simulink model "woutModel"  (R2019b)
settings: Solver=VariableStepAuto  StartTime=0.0  StopTime=10.0  RelTol=1e-3
model workspace (MAT data in the model file):
  I1 = 0.074
  I2 = 0.00012
  L = 0.6
  P1 = 0.4356
  P2 = 0.00372
  P3 = 0.036
  Sig = Simulink.Signal
  Sig.DataType = 'auto'
  Sig.Dimensions = -1
  Sig.DimensionsMode = 'auto'
  Sig.Complexity = 'auto'
  Sig.SampleTime = -1
  Sig.SamplingMode = 'auto'
  b1 = 4.8
  b2 = 0.0002
  c1 = 0.04
  c2 = 0.06
  ddtheta = sym
  ddtheta.s = 'symobj::fromString("eJzNVktv1DAQdjYppRTKHkDlUUSg3HqBHouQUm2ptIeKAxdukZc4W6PESeMsND31yC/gP8FvQlpsJ0u8tuPsIg6NNIpnMpnHN4/EBQAMALj+we6e62ywW/AE1JfLzg+aM9MBW5xoRSGleEqEeOn5IadvCBeR/xUWGE4S5BOYIurPKIp8THxapdnky8ksTatxhEiJY4wKIPscKDY9TudZEik6XTEKfZpkpSK/xYmWUYInwt8d0F73OFFUfqzS4wRDimid22PJxy9J/78B9pBTJyargfKqkTNZsN+cHQWkfwHM5XSSpSpYAsgzWBb4UsTY5dNVzj8lG57Cbyg+7nN6f5kXiAGXkVOMeKogeNraE76ft/a4f489D3ZaM0s2eU4DHAm57HvbYOeMyVygXdp7Mn/X0jCuEssmp1FGSlZubvdFIx8y+l7HACJLzW5zChEDiKILU90+zIRdrc4RLKEhj4Ufz2QrxDGw6NSxJPCqCrPCErPomxBdzGAisJTxdZzmbpLP2WXppd2+OSFZzuY52FvY7LDzqG+O6xwhES3UV5sENZlqPmT+mSUv36C7mPWBYe7k/uJ9NKyX3dHRmMSY4LLqmcdVl6XIT7Jpw9DmT62HmoOIYQTzPKlEDKvukgOjHRzVo9bdK4KyXPOlzUMKuVKw28a/ZFOO5bXC7xli7drR6+Qo9gmr1+mMfAY9Prd7/GiYGHbmsGcX3gRexqfefTiO5V07n1/Lu1bOm8ucGGh5q9jp+7X20YWv2g8Hlvkx7jJYTGnvji0gmSIR+9IuHTR3S78eK/zOmr0j828V/t0N6Im1e6ascqTo8e98z3+I87vHtqgTpleoyMT7q/yP9NVF5rl+17+Io+iODe921XjLUGOt/6S8uvpsU3qmxqP6GBlmRN69L9tY/87uou8bXv8+R1F5jkp4aHn2xjR/++Gn8A82IAgb", 2)'
  ddtheta.digits = 32
  ddtheta1 = sym
  ddtheta1.s = 'symobj::fromString("eJytkEEKwjAQRce2igrudKGrXEFPoODGtSdIyWgjSQqdVMnOU3goT2XSCsZCwYUDjxkmn/zkpwCQANwfvmfpYOjbdgVtpX6ev2evgUmAHHEieTbN+ut8E7ihrAS78kryXCEzXCOxmlAwaRg5XeaXfa21Owg0Vp4kVhB7Jp07s0BRKtHR9L2x0ZMqbWc/CpAVSuaN3xQ+NQsQ2qPTOyU5IbV/W0Yez0j/t8AWgd5Mfgsl3o8DQtgCLV+/AARuPcI=", 2)'
  ddtheta1.digits = 32
  ddtheta2 = sym
  ddtheta2.s = 'symobj::fromString("eJytkEEKwjAQRce2igrudKGrnKEnUHDj2hOkZLSRJIVOqmTnKTyUpzJpBWOh4MKBxwyTT37yUwBIAO4P37N0NPZtu4GuUj8v37PXwCxAjjiRPJt2/XWeB24oa8GuvJa8UMgM10isIRRMGkZOV8Vl32jtDgKNlSeJNcSeSe/OLFBWSvQ0Q29s9aQq29tPAmSFkkXrN4dPLQKE9uj0TklOSN3f1pHHM9L/LbBVYDCT30KJ99OAELZEy/MXBG89w3==", 2)'
  ddtheta2.digits = 32
  dtheta = sym
  dtheta.s = 'symobj::fromString("eJzNV09v0zAUd5qOMQajB9D4M0Rgu+0CHIeQMnVM6mHiwIVb5BKnM0qcLHZh2WlHPgHfCT4TUrGdlDiOnbSIwyI9Je/55ff+v6YuAGAAwPUPfh+6zga/+U9Aebn8+UH1zHXAliBaUEgpnhEpbpy/EfQN4Tz0vsIcw2mMPAITRL05RaGHiUeLJJ1+OZknSTEJEWE4wigHqs2BhjkUdJ7GoaZj81Hq0zhlmvyWIMrCGE+lvTugvu4Jooh9LJLjGEOKaBnbY8XGL0X/vyXsoSBrTlZLykEl5zJ/v3p2tCT9S8JcQSdpoidLJvIMshxfSh9tNl3t+aeCMdT4Dc3GfUHvL7Mc8cSl5BQjESrwn9Z40vbzGk/YH/Jzf6eGaWCKmAY4lHLV9rYB54zLXNC6Wu+p/N2OhnE1XzYFjVPCeLkF7otKPuL0vfQBhB01uy0oQDxBFF2Y6vZhLnFbdQ4hg4Y4lnaGJqwAR6BDp/QlhldFkOYdPsu+CdDFHMYyl2p+Hae6m+QLfnX00m7fnJA04/Ps7y0xLTiP+ua4jBES2UJ9tYlRFWnLhso/64jLM+guZ31gmDu1v0Qfjcpld3Q0IREmmBU987jqspTxKZhdOeyyp9dDj0H6MIZZFhfSh1V3yaERB4flqNl7RVKatWy15iGBQsnfrf1vYKq+vNL4PYOvth29Toxyn/B6nc7JZ9Bjc7vHTisnhp056tmFN4FX81PuPhxF6q5dLK7VXavGLWROBFpx67lr79fShi2/ej8cdsyPcZfBfEZ7d2wOyQxJ3xu7dFDdO/r1WON31uwdlX+r8e9uQE+s3TOsyJCmJ37ne75DnN892LJOmF6hPJXvr/I90lcXlRf6tm8RR9OdGN611XjLUONW/ylx2fpsUznT/dFtjA0zou7el7Wvf2d32fcV3/BR7sqQnSMGxf8V29lr/Uz2w37wKfgDFsMHTw==", 2)'
  dtheta.digits = 32
  dtheta1 = sym
  dtheta1.s = 'symobj::fromString("eJytkEEKwjAQRce2KgrudKGrXEFPoODGtSdIyWgjSQqdVMnOU3goT2XSCsZCwYUDjxkmn/zkpwCQANwfvmfpYOjbdgVtpX6ev2evgUmAHHEieTbN+ut8E7ihrAS78kryXCEzXCOxmlAwaRg5XeaXfa21Owg0Vp4kVhB7Jp07s0BRKtHR9L2x0ZMqbWc/CpAVSuaN3xQ+NQsQ2qPTOyU5IbV/W0Yez0j/t8AWgd5Mfgsl3o8DwhZo+RpeA+M9XH==", 2)'
  dtheta1.digits = 32
  dtheta2 = sym
  dtheta2.s = 'symobj::fromString("eJytkEEKwjAQRce2KgrudKGrnKEnUHDj2hOkZLSRJIVOqmTnKTyUpzJpBWOh4MKBxwyTT37yUwBIAO4P37N0NPZtu4GuUj8v37PXwCxAjjiRPJt2/XWeB24oa8GuvJa8UMgM10isIRRMGkZOV8Vl32jtDgKNlSeJNcSeSe/OLFBWSvQ0Q29s9aQq29tPAmSFkkXrN4dPLQKE9uj0TklOSN3f1pHHM9L/LbBVYDCT30KJ99OAsCVansMLA+U9XX==", 2)'
  dtheta2.digits = 32
  g = 9.81
  g1 = 6.2784
  g2 = 0.5886
  k_m = 50
  l1 = 0.6
  m1 = 1
  m2 = 1
  tau_e = 0.03
  theta = sym
  theta.s = 'symobj::fromString("eJzNVs1u1DAQdjYppRTKHkDlp4hAufUCPRYhpdpSaQ8VBy7cIi9xtkaJk8ZeaHrqkSfgneCZkBbbyRKv7SS7iEMjjZIZT+b3m0lcAMAAgOsf/O65zga/BU9Adbn8+UH9zHXAliBaUkgpnhIpXjo/FPQN4SLyv8ICw0mCfAJTRP0ZRZGPiU/LNJt8OZmlaTmOEGE4xqgAqs+BZtMTdJ4lkabTFqPUp0nGNPktQZRFCZ5If3dAc90TRBH7WKbHCYYU0Sq3x4qPX4r+fyvYQ0GtNVmtKK9qOZcF+/WzoxXpXwrmCjrJUr1YspBnkBX4UsbY5tPVnn8qNjyN39B83Bf0/jIvEC9cRk4xEqmC4GljT/p+3tgT/j1+Huw0ZpZsipwGOJJy1fe2xc4Zl7nAuIz3VP5uB2BcLZZNQaOMMN5uYfdFLR9y+l7FAKKOnt0WFCJeIIoubH37MJN2jT5HkEFLHgs/ns1WiGPQoVPFksCrMsyKjpglbkJ0MYOJrKVaX8ep7zb5nF8dWNrtmxOS5Xyeg72FzRY7j/rmuMoREgmhvt4kqM7U8KHyzzry8i26i1kfWOZOxZfA0bBadkdHYxJjglnZM4+rLkuZn2Kzq4Zd/vR+6DnIGEYwz5NSxrDqLjmw2sFRNWrtWJGU5YYvYx5SKJSC3Sb+JZtqLK81fs8Sa9uOXidHuU94v05n5DPo8bnd48eoiWVnDnt24U3g1fpUuw/Hsbpr5/NrddeqeQuZEwMjb7125n6tfLTVV8fDQcf8WHcZLKa0d8cWkEyRjH1plw7qewdejzV+Z03sqPxbjX93AzCxNmZYmSNNT3zne/5DnN89tmWfML1CRSbfX+V/pK8vKi/02/5FHE13bHm3rcdblh4b+FPyasPZpnKmx6P7GFlmRN29L5tY/87uAvc1b8bIzhGDhzJG+9kb40ziYT/8FP4B9o8Ggw==", 2)'
  theta.digits = 32
  theta1 = sym
  theta1.s = 'symobj::fromString("eJytkMEKwjAMhuM2BQVvetBTX0GfQMGLZ5+go9FF2g6WTtnNp/ChfCrbTXBOBh4MfCSkP0nzxwAQAdzuPifxYOjTZglNxL6evWqvgXGAK5bMdLJ1++N9HbgiFUpcZEEy1SisNMiiZFSCrODK5Ol5VxpT7RVaR0fCAto7o87MJJDlWnU0fX+s9axz1+mPAuyUprTeN4F3TAOM7lCZrSbJyM1ti9aOR0v/N8PmgV5PfjPl60iXoZMrgCcC9Dz2", 2)'
  theta1.digits = 32
  theta2 = sym
  theta2.s = 'symobj::fromString("eJxjZmBgYGJgaJgGpFmYGVmBlIMUAwQwA9kiUDZQDQMnCBdXFicWF2em54GFUeSNQLg8NbMoRaEssSgzMSknVSEvMTe1WKG0ODVFITNPobgyNz8py6U0N7fSMyU1ryQzLTO1iAHZTiY0M1lAOCM/JwVNDS43gtUX5+SXoImzgXBxSUpOZhLYPi4GBOAF4eLUkuDKXMeczMTi1GKI3ySR7DiFpJ5qASYKwjjDhLhAwfBkSUZqSSIwKgAC9zz3", 2)'
  theta2.digits = 32
  u = sym
  u.s = 'symobj::fromString("eJxjZmBgYGJgaJgGpFmYGVmBlIMUAwQwA9kiUDZQDQMnCBdXFicWF2em54GFUeSNQLg8NbMoRaEssSgzMSknVSEvMTe1WKG0ODVFITNPobgyNz8py6U0N7fSMyU1ryQzLTO1iAHZTiY0M1lAOCM/JwVNDS43gtUX5+SXoImzgXBxSUpOZhLYPi4GBOAF4eLUkuDKXMeczMTi1GKI3ySR7DiFpJ5qASYKwjjDhLhAQRZnBOFSIAEADIY7Gt==", 2)'
  u.digits = 32
settings Model: Creator=houte  LastModifiedBy=houte
settings DataIOCC: LoadExternalInput=on

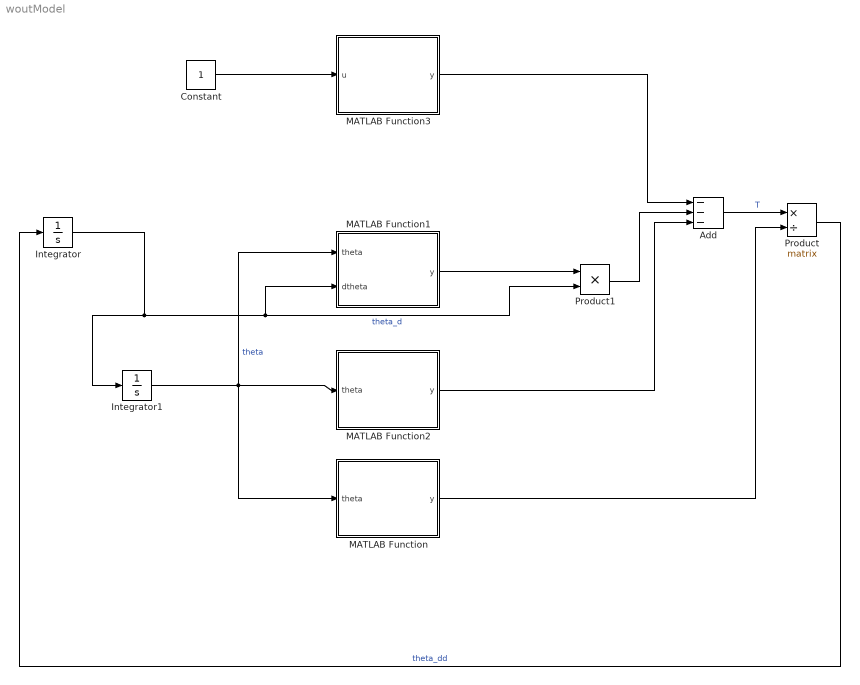
== system woutModel ==
  Add : Sum  Inputs=---
  Constant : Constant
  Integrator : Integrator  InitialCondition=[0; 0]
  Integrator1 : Integrator  InitialCondition=[0;0]
  MATLAB Function : MATLAB Function  TreatAsAtomicUnit=on
  MATLAB Function1 : MATLAB Function  TreatAsAtomicUnit=on
  MATLAB Function2 : MATLAB Function  TreatAsAtomicUnit=on
  MATLAB Function3 : MATLAB Function  TreatAsAtomicUnit=on
  Product : Product  Inputs=*/  Multiplication=Matrix(*)
  Product1 : Product
  wires:
  Integrator/1 -> Product1/2, MATLAB Function1/2(dtheta), Integrator1/1  "theta_d"
  Integrator1/1 -> MATLAB Function1/1(theta), MATLAB Function/1(theta), MATLAB Function2/1(theta)  "theta"
  Product1/1 -> Add/2
  Add/1 -> Product/1  "T"
  MATLAB Function1/1(y) -> Product1/1
  MATLAB Function3/1(y) -> Add/1
  MATLAB Function2/1(y) -> Add/3
  MATLAB Function/1(y) -> Product/2
  Product/1 -> Integrator/1  "theta_dd"
  Constant/1 -> MATLAB Function3/1(u)

== matlab function woutModel/MATLAB Function1 ==
  data: theta input; y output; dtheta input
function y = C(theta, dtheta)
    theta1 = theta(1);
    theta2 = theta(2);
    dtheta1 = dtheta(1);
    dtheta2 = dtheta(2);


y = [b1 - P3*dtheta2*sin(theta2), -P3*(dtheta1+dtheta2)*sin(theta2);
    P3*dtheta1*sin(theta2), b2];

== matlab function woutModel/MATLAB Function ==
  data: theta input; y output
function y = M(theta)
theta1 = theta(1);
theta2 = theta(2);

y = [P1 + P2 + 2*P3*cos(theta2), P2 + P3 * cos(theta2);
     P2 + P3*cos(theta2), P2];

== matlab function woutModel/MATLAB Function2 ==
  data: theta input; y output; g1 parameter
function y = G(theta,g1)

    g1 = 6.278400000000000;
    g2 = 0.588600000000000;
    theta1 = theta(1);
    theta2 = theta(2);

y = [-g1*sin(theta1) - g2*sin(theta1+theta2);
     -g2*sin(theta1+theta2)];

== matlab function woutModel/MATLAB Function3 ==
  data: u input; y output
function y = T(u)
    km =1;
    % T = km*u - Te*dTe;
    T = km*u;

y = [T; 0];
